simulink model "c00019M_harness"  (R2018a)
settings: Solver=ode3  StartTime=0.0  StopTime=10.0  RelTol=1e-3  EnableMultiTasking=on
undefined symbols (not defined in the file): b, DiscIntNeverNeededParam, J, K, L, PosMinimaW4, R, sigbuilder_block
(part 2 of 3)

== system c00019M_harness/CPSUT/Cyber/WL1 ==
  note: Sensors
  WPos : Inport
  User : Inport  Port=2
  OW : Inport  Port=3
  Chart1 : Stateflow chart  TreatAsAtomicUnit=on
  Constant : Constant  Value=-1
  Data Type Conversion : DataTypeConversion
  Switch : Switch  Criteria=u2 ~= 0  Threshold=1  ZeroCross=off
  WindowLogicOutput : Outport
  wires:
  Data Type Conversion/1 -> Switch/2
  Constant/1 -> Switch/1
  User/1 -> Chart1/2(UI)
  WPos/1 -> Chart1/1(S)
  Switch/1 -> WindowLogicOutput/1
  OW/1 -> Data Type Conversion/1
  Chart1/1(W) -> Switch/3

== system c00019M_harness/CPSUT/Cyber/WL3 ==
  note: Sensors
  WPos : Inport
  User : Inport  Port=2
  OW : Inport  Port=3
  L : Inport  Port=4
  Chart2 : Stateflow chart  TreatAsAtomicUnit=on
  Constant : Constant  Value=-1
  Constant1 : Constant  Value=0
  Constant2 : Constant  Value=PosMinimaW4
  Data Type Conversion : DataTypeConversion
  Switch : Switch  Criteria=u2 ~= 0  Threshold=1  ZeroCross=off
  Switch1 : Switch  Criteria=u2 ~= 0
  WindowLogicOutput : Outport
  wires:
  L/1 -> Switch1/2
  Data Type Conversion/1 -> Switch/2
  Constant/1 -> Switch/1
  Chart2/1(W) -> Switch1/3
  User/1 -> Chart2/2(UI)
  WPos/1 -> Chart2/1(S)
  Switch1/1 -> Switch/3
  Constant1/1 -> Switch1/1
  Switch/1 -> WindowLogicOutput/1
  OW/1 -> Data Type Conversion/1
  Constant2/1 -> Chart2/3(PosMinW4)

== system c00019M_harness/CPSUT/Physical/W ==
  WIn : Inport
  DC_Engine : Subsystem
  Discrete-Time Integrator : DiscreteIntegrator  InitialCondition=5  SampleTime=-1  LimitOutput=on  UpperSaturationLimit=5  LowerSaturationLimit=0  ICPrevOutput=DiscIntNeverNeededParam  ICPrevScaledInput=DiscIntNeverNeededParam
  WPos : Outport
  wires:
  Discrete-Time Integrator/1 -> WPos/1
  DC_Engine/1(Speed) -> Discrete-Time Integrator/1
  WIn/1 -> DC_Engine/1(input)

== system c00019M_harness/CPSUT/Physical/W5 ==
  WIn : Inport
  DC_Engine : Subsystem
  Discrete-Time Integrator : DiscreteIntegrator  InitialCondition=5  SampleTime=-1  LimitOutput=on  UpperSaturationLimit=5  LowerSaturationLimit=0  ICPrevOutput=DiscIntNeverNeededParam  ICPrevScaledInput=DiscIntNeverNeededParam
  WPos : Outport
  wires:
  WIn/1 -> DC_Engine/1(input)
  DC_Engine/1(Speed) -> Discrete-Time Integrator/1
  Discrete-Time Integrator/1 -> WPos/1

== system c00019M_harness/CPSUT/Physical/W7 ==
  WIn : Inport
  DC_Engine : Subsystem
  Discrete-Time Integrator : DiscreteIntegrator  InitialCondition=5  SampleTime=-1  LimitOutput=on  UpperSaturationLimit=5  LowerSaturationLimit=PosMinimaW4  ICPrevOutput=DiscIntNeverNeededParam  ICPrevScaledInput=DiscIntNeverNeededParam
  WPos : Outport
  wires:
  WIn/1 -> DC_Engine/1(input)
  DC_Engine/1(Speed) -> Discrete-Time Integrator/1
  Discrete-Time Integrator/1 -> WPos/1

== system c00019M_harness/M004/Cyber/Pri ==
  P : Inport
  CW2C : Inport  Port=2
  Switch1 : Switch  Criteria=u2 > Threshold  Threshold=4
  User : Outport
  wires:
  CW2C/1 -> Switch1/3
  P/1 -> Switch1/1, Switch1/2
  Switch1/1 -> User/1

== system c00019M_harness/M004/Cyber/Pri3 ==
  D : Inport
  CW1C : Inport  Port=2
  Switch : Switch  Criteria=u2 ~= 0
  User : Outport
  wires:
  D/1 -> Switch/1, Switch/2
  Switch/1 -> User/1
  CW1C/1 -> Switch/3

== system c00019M_harness/M004/Cyber/Pri4 ==
  P : Inport
  CW4C : Inport  Port=2
  Switch1 : Switch  Criteria=u2 ~= 0
  User : Outport
  wires:
  P/1 -> Switch1/1, Switch1/2
  CW4C/1 -> Switch1/3
  Switch1/1 -> User/1

== system c00019M_harness/M004/Cyber/WL ==
  note: Sensors
  WPos : Inport
  User : Inport  Port=2
  OW : Inport  Port=3
  Chart : Stateflow chart  TreatAsAtomicUnit=on
  Constant : Constant  Value=-1
  Data Type Conversion : DataTypeConversion
  Switch : Switch  Criteria=u2 ~= 0  Threshold=1  ZeroCross=off
  WindowLogicOutput : Outport
  wires:
  Data Type Conversion/1 -> Switch/2
  Constant/1 -> Switch/1
  User/1 -> Chart/2(UI)
  WPos/1 -> Chart/1(S)
  Switch/1 -> WindowLogicOutput/1
  OW/1 -> Data Type Conversion/1
  Chart/1(W) -> Switch/3

== system c00019M_harness/M004/Cyber/WL1 ==
  note: Sensors
  WPos : Inport
  User : Inport  Port=2
  OW : Inport  Port=3
  Chart1 : Stateflow chart  TreatAsAtomicUnit=on
  Constant : Constant  Value=-1
  Data Type Conversion : DataTypeConversion
  Switch : Switch  Criteria=u2 ~= 0  Threshold=1  ZeroCross=off
  WindowLogicOutput : Outport
  wires:
  OW/1 -> Data Type Conversion/1
  Switch/1 -> WindowLogicOutput/1
  WPos/1 -> Chart1/1(S)
  User/1 -> Chart1/2(UI)
  Constant/1 -> Switch/1
  Data Type Conversion/1 -> Switch/2
  Chart1/1(W) -> Switch/3

== system c00019M_harness/M004/Cyber/WL3 ==
  note: Sensors
  WPos : Inport
  User : Inport  Port=2
  OW : Inport  Port=3
  L : Inport  Port=4
  Chart2 : Stateflow chart  TreatAsAtomicUnit=on
  Constant : Constant  Value=-1
  Constant1 : Constant  Value=0
  Constant2 : Constant  Value=PosMinimaW4
  Data Type Conversion : DataTypeConversion
  Switch : Switch  Criteria=u2 ~= 0  Threshold=1  ZeroCross=off
  Switch1 : Switch  Criteria=u2 ~= 0
  WindowLogicOutput : Outport
  wires:
  Constant2/1 -> Chart2/3(PosMinW4)
  OW/1 -> Data Type Conversion/1
  Switch/1 -> WindowLogicOutput/1
  Constant1/1 -> Switch1/1
  Switch1/1 -> Switch/3
  WPos/1 -> Chart2/1(S)
  User/1 -> Chart2/2(UI)
  Chart2/1(W) -> Switch1/3
  Constant/1 -> Switch/1
  Data Type Conversion/1 -> Switch/2
  L/1 -> Switch1/2

== system c00019M_harness/M004/Physical/W ==
  WIn : Inport
  DC_Engine : Subsystem
  Discrete-Time Integrator : DiscreteIntegrator  InitialCondition=5  SampleTime=-1  LimitOutput=on  UpperSaturationLimit=5  LowerSaturationLimit=0  ICPrevOutput=DiscIntNeverNeededParam  ICPrevScaledInput=DiscIntNeverNeededParam
  WPos : Outport
  wires:
  WIn/1 -> DC_Engine/1(input)
  DC_Engine/1(Speed) -> Discrete-Time Integrator/1
  Discrete-Time Integrator/1 -> WPos/1

== system c00019M_harness/M004/Physical/W5 ==
  WIn : Inport
  DC_Engine : Subsystem
  Discrete-Time Integrator : DiscreteIntegrator  InitialCondition=5  SampleTime=-1  LimitOutput=on  UpperSaturationLimit=5  LowerSaturationLimit=0  ICPrevOutput=DiscIntNeverNeededParam  ICPrevScaledInput=DiscIntNeverNeededParam
  WPos : Outport
  wires:
  Discrete-Time Integrator/1 -> WPos/1
  DC_Engine/1(Speed) -> Discrete-Time Integrator/1
  WIn/1 -> DC_Engine/1(input)

== system c00019M_harness/M004/Physical/W7 ==
  WIn : Inport
  DC_Engine : Subsystem
  Discrete-Time Integrator : DiscreteIntegrator  InitialCondition=5  SampleTime=-1  LimitOutput=on  UpperSaturationLimit=5  LowerSaturationLimit=PosMinimaW4  ICPrevOutput=DiscIntNeverNeededParam  ICPrevScaledInput=DiscIntNeverNeededParam
  WPos : Outport
  wires:
  Discrete-Time Integrator/1 -> WPos/1
  DC_Engine/1(Speed) -> Discrete-Time Integrator/1
  WIn/1 -> DC_Engine/1(input)

== system c00019M_harness/M014/Cyber/Pri ==
  P : Inport
  CW2C : Inport  Port=2
  Switch1 : Switch  Criteria=u2 ~= 0
  User : Outport
  wires:
  CW2C/1 -> Switch1/3
  P/1 -> Switch1/1, Switch1/2
  Switch1/1 -> User/1

== system c00019M_harness/M014/Cyber/Pri3 ==
  D : Inport
  CW1C : Inport  Port=2
  Switch : Switch  Criteria=u2 > Threshold  Threshold=4
  User : Outport
  wires:
  D/1 -> Switch/1, Switch/2
  Switch/1 -> User/1
  CW1C/1 -> Switch/3

== system c00019M_harness/M014/Cyber/Pri4 ==
  P : Inport
  CW4C : Inport  Port=2
  Switch1 : Switch  Criteria=u2 ~= 0
  User : Outport
  wires:
  P/1 -> Switch1/1, Switch1/2
  CW4C/1 -> Switch1/3
  Switch1/1 -> User/1

== system c00019M_harness/M014/Cyber/WL ==
  note: Sensors
  WPos : Inport
  User : Inport  Port=2
  OW : Inport  Port=3
  Chart : Stateflow chart  TreatAsAtomicUnit=on
  Constant : Constant  Value=-1
  Data Type Conversion : DataTypeConversion
  Switch : Switch  Criteria=u2 ~= 0  Threshold=1  ZeroCross=off
  WindowLogicOutput : Outport
  wires:
  Data Type Conversion/1 -> Switch/2
  Constant/1 -> Switch/1
  User/1 -> Chart/2(UI)
  WPos/1 -> Chart/1(S)
  Switch/1 -> WindowLogicOutput/1
  OW/1 -> Data Type Conversion/1
  Chart/1(W) -> Switch/3

== system c00019M_harness/M014/Cyber/WL1 ==
  note: Sensors
  WPos : Inport
  User : Inport  Port=2
  OW : Inport  Port=3
  Chart1 : Stateflow chart  TreatAsAtomicUnit=on
  Constant : Constant  Value=-1
  Data Type Conversion : DataTypeConversion
  Switch : Switch  Criteria=u2 ~= 0  Threshold=1  ZeroCross=off
  WindowLogicOutput : Outport
  wires:
  OW/1 -> Data Type Conversion/1
  Switch/1 -> WindowLogicOutput/1
  WPos/1 -> Chart1/1(S)
  User/1 -> Chart1/2(UI)
  Constant/1 -> Switch/1
  Data Type Conversion/1 -> Switch/2
  Chart1/1(W) -> Switch/3

== system c00019M_harness/M014/Cyber/WL3 ==
  note: Sensors
  WPos : Inport
  User : Inport  Port=2
  OW : Inport  Port=3
  L : Inport  Port=4
  Chart2 : Stateflow chart  TreatAsAtomicUnit=on
  Constant : Constant  Value=-1
  Constant1 : Constant  Value=0
  Constant2 : Constant  Value=PosMinimaW4
  Data Type Conversion : DataTypeConversion
  Switch : Switch  Criteria=u2 ~= 0  Threshold=1  ZeroCross=off
  Switch1 : Switch  Criteria=u2 ~= 0
  WindowLogicOutput : Outport
  wires:
  Constant2/1 -> Chart2/3(PosMinW4)
  OW/1 -> Data Type Conversion/1
  Switch/1 -> WindowLogicOutput/1
  Constant1/1 -> Switch1/1
  Switch1/1 -> Switch/3
  WPos/1 -> Chart2/1(S)
  User/1 -> Chart2/2(UI)
  Chart2/1(W) -> Switch1/3
  Constant/1 -> Switch/1
  Data Type Conversion/1 -> Switch/2
  L/1 -> Switch1/2

== system c00019M_harness/M014/Physical/W ==
  WIn : Inport
  DC_Engine : Subsystem
  Discrete-Time Integrator : DiscreteIntegrator  InitialCondition=5  SampleTime=-1  LimitOutput=on  UpperSaturationLimit=5  LowerSaturationLimit=0  ICPrevOutput=DiscIntNeverNeededParam  ICPrevScaledInput=DiscIntNeverNeededParam
  WPos : Outport
  wires:
  WIn/1 -> DC_Engine/1(input)
  DC_Engine/1(Speed) -> Discrete-Time Integrator/1
  Discrete-Time Integrator/1 -> WPos/1

== system c00019M_harness/M014/Physical/W5 ==
  WIn : Inport
  DC_Engine : Subsystem
  Discrete-Time Integrator : DiscreteIntegrator  InitialCondition=5  SampleTime=-1  LimitOutput=on  UpperSaturationLimit=5  LowerSaturationLimit=0  ICPrevOutput=DiscIntNeverNeededParam  ICPrevScaledInput=DiscIntNeverNeededParam
  WPos : Outport
  wires:
  Discrete-Time Integrator/1 -> WPos/1
  DC_Engine/1(Speed) -> Discrete-Time Integrator/1
  WIn/1 -> DC_Engine/1(input)

== system c00019M_harness/M014/Physical/W7 ==
  WIn : Inport
  DC_Engine : Subsystem
  Discrete-Time Integrator : DiscreteIntegrator  InitialCondition=5  SampleTime=-1  LimitOutput=on  UpperSaturationLimit=5  LowerSaturationLimit=PosMinimaW4  ICPrevOutput=DiscIntNeverNeededParam  ICPrevScaledInput=DiscIntNeverNeededParam
  WPos : Outport
  wires:
  Discrete-Time Integrator/1 -> WPos/1
  DC_Engine/1(Speed) -> Discrete-Time Integrator/1
  WIn/1 -> DC_Engine/1(input)

== system c00019M_harness/M018/Cyber/Pri ==
  P : Inport
  CW2C : Inport  Port=2
  Switch1 : Switch  Criteria=u2 ~= 0
  User : Outport
  wires:
  CW2C/1 -> Switch1/3
  P/1 -> Switch1/1, Switch1/2
  Switch1/1 -> User/1

== system c00019M_harness/M018/Cyber/Pri3 ==
  D : Inport
  CW1C : Inport  Port=2
  Switch : Switch  Criteria=u2 ~= 0
  User : Outport
  wires:
  D/1 -> Switch/1, Switch/2
  Switch/1 -> User/1
  CW1C/1 -> Switch/3

== system c00019M_harness/M018/Cyber/Pri4 ==
  P : Inport
  CW4C : Inport  Port=2
  Switch1 : Switch  Criteria=u2 > Threshold  Threshold=4
  User : Outport
  wires:
  P/1 -> Switch1/1, Switch1/2
  CW4C/1 -> Switch1/3
  Switch1/1 -> User/1

== system c00019M_harness/M018/Cyber/WL ==
  note: Sensors
  WPos : Inport
  User : Inport  Port=2
  OW : Inport  Port=3
  Chart : Stateflow chart  TreatAsAtomicUnit=on
  Constant : Constant  Value=-1
  Data Type Conversion : DataTypeConversion
  Switch : Switch  Criteria=u2 ~= 0  Threshold=1  ZeroCross=off
  WindowLogicOutput : Outport
  wires:
  Data Type Conversion/1 -> Switch/2
  Constant/1 -> Switch/1
  User/1 -> Chart/2(UI)
  WPos/1 -> Chart/1(S)
  Switch/1 -> WindowLogicOutput/1
  OW/1 -> Data Type Conversion/1
  Chart/1(W) -> Switch/3

== system c00019M_harness/M018/Cyber/WL1 ==
  note: Sensors
  WPos : Inport
  User : Inport  Port=2
  OW : Inport  Port=3
  Chart1 : Stateflow chart  TreatAsAtomicUnit=on
  Constant : Constant  Value=-1
  Data Type Conversion : DataTypeConversion
  Switch : Switch  Criteria=u2 ~= 0  Threshold=1  ZeroCross=off
  WindowLogicOutput : Outport
  wires:
  OW/1 -> Data Type Conversion/1
  Switch/1 -> WindowLogicOutput/1
  WPos/1 -> Chart1/1(S)
  User/1 -> Chart1/2(UI)
  Constant/1 -> Switch/1
  Data Type Conversion/1 -> Switch/2
  Chart1/1(W) -> Switch/3

== system c00019M_harness/M018/Cyber/WL3 ==
  note: Sensors
  WPos : Inport
  User : Inport  Port=2
  OW : Inport  Port=3
  L : Inport  Port=4
  Chart2 : Stateflow chart  TreatAsAtomicUnit=on
  Constant : Constant  Value=-1
  Constant1 : Constant  Value=0
  Constant2 : Constant  Value=PosMinimaW4
  Data Type Conversion : DataTypeConversion
  Switch : Switch  Criteria=u2 ~= 0  Threshold=1  ZeroCross=off
  Switch1 : Switch  Criteria=u2 ~= 0
  WindowLogicOutput : Outport
  wires:
  Constant2/1 -> Chart2/3(PosMinW4)
  OW/1 -> Data Type Conversion/1
  Switch/1 -> WindowLogicOutput/1
  Constant1/1 -> Switch1/1
  Switch1/1 -> Switch/3
  WPos/1 -> Chart2/1(S)
  User/1 -> Chart2/2(UI)
  Chart2/1(W) -> Switch1/3
  Constant/1 -> Switch/1
  Data Type Conversion/1 -> Switch/2
  L/1 -> Switch1/2

== system c00019M_harness/M018/Physical/W ==
  WIn : Inport
  DC_Engine : Subsystem
  Discrete-Time Integrator : DiscreteIntegrator  InitialCondition=5  SampleTime=-1  LimitOutput=on  UpperSaturationLimit=5  LowerSaturationLimit=0  ICPrevOutput=DiscIntNeverNeededParam  ICPrevScaledInput=DiscIntNeverNeededParam
  WPos : Outport
  wires:
  WIn/1 -> DC_Engine/1(input)
  DC_Engine/1(Speed) -> Discrete-Time Integrator/1
  Discrete-Time Integrator/1 -> WPos/1

== system c00019M_harness/M018/Physical/W5 ==
  WIn : Inport
  DC_Engine : Subsystem
  Discrete-Time Integrator : DiscreteIntegrator  InitialCondition=5  SampleTime=-1  LimitOutput=on  UpperSaturationLimit=5  LowerSaturationLimit=0  ICPrevOutput=DiscIntNeverNeededParam  ICPrevScaledInput=DiscIntNeverNeededParam
  WPos : Outport
  wires:
  Discrete-Time Integrator/1 -> WPos/1
  DC_Engine/1(Speed) -> Discrete-Time Integrator/1
  WIn/1 -> DC_Engine/1(input)

== system c00019M_harness/M018/Physical/W7 ==
  WIn : Inport
  DC_Engine : Subsystem
  Discrete-Time Integrator : DiscreteIntegrator  InitialCondition=5  SampleTime=-1  LimitOutput=on  UpperSaturationLimit=5  LowerSaturationLimit=PosMinimaW4  ICPrevOutput=DiscIntNeverNeededParam  ICPrevScaledInput=DiscIntNeverNeededParam
  WPos : Outport
  wires:
  Discrete-Time Integrator/1 -> WPos/1
  DC_Engine/1(Speed) -> Discrete-Time Integrator/1
  WIn/1 -> DC_Engine/1(input)

== system c00019M_harness/M028/Cyber/Pri ==
  P : Inport
  CW2C : Inport  Port=2
  Switch1 : Switch  Criteria=u2 ~= 0
  User : Outport
  wires:
  CW2C/1 -> Switch1/3
  P/1 -> Switch1/1, Switch1/2
  Switch1/1 -> User/1

== system c00019M_harness/M028/Cyber/Pri3 ==
  D : Inport
  CW1C : Inport  Port=2
  Switch : Switch  Criteria=u2 ~= 0
  User : Outport
  wires:
  D/1 -> Switch/1, Switch/2
  Switch/1 -> User/1
  CW1C/1 -> Switch/3

== system c00019M_harness/M028/Cyber/Pri4 ==
  P : Inport
  CW4C : Inport  Port=2
  Switch1 : Switch  Criteria=u2 ~= 0
  User : Outport
  wires:
  P/1 -> Switch1/1, Switch1/2
  CW4C/1 -> Switch1/3
  Switch1/1 -> User/1

== system c00019M_harness/M028/Cyber/WL ==
  note: Sensors
  WPos : Inport
  User : Inport  Port=2
  OW : Inport  Port=3
  Chart : Stateflow chart  TreatAsAtomicUnit=on
  Constant : Constant  Value=-1
  Data Type Conversion : DataTypeConversion
  Switch : Switch  Criteria=u2 ~= 0  Threshold=1  ZeroCross=off
  WindowLogicOutput : Outport
  wires:
  Data Type Conversion/1 -> Switch/2
  Constant/1 -> Switch/1
  User/1 -> Chart/2(UI)
  WPos/1 -> Chart/1(S)
  Switch/1 -> WindowLogicOutput/1
  OW/1 -> Data Type Conversion/1
  Chart/1(W) -> Switch/3

== system c00019M_harness/M028/Cyber/WL1 ==
  note: Sensors
  WPos : Inport
  User : Inport  Port=2
  OW : Inport  Port=3
  Chart1 : Stateflow chart  TreatAsAtomicUnit=on
  Constant : Constant  Value=-1
  Data Type Conversion : DataTypeConversion
  Switch : Switch  Criteria=u2 ~= 0  Threshold=1  ZeroCross=off
  WindowLogicOutput : Outport
  wires:
  OW/1 -> Data Type Conversion/1
  Switch/1 -> WindowLogicOutput/1
  WPos/1 -> Chart1/1(S)
  User/1 -> Chart1/2(UI)
  Constant/1 -> Switch/1
  Data Type Conversion/1 -> Switch/2
  Chart1/1(W) -> Switch/3

== system c00019M_harness/M028/Cyber/WL3 ==
  note: Sensors
  WPos : Inport
  User : Inport  Port=2
  OW : Inport  Port=3
  L : Inport  Port=4
  Chart2 : Stateflow chart  TreatAsAtomicUnit=on
  Constant : Constant  Value=-1
  Constant1 : Constant  Value=0
  Constant2 : Constant  Value=PosMinimaW4
  Data Type Conversion : DataTypeConversion
  Switch : Switch  Criteria=u2 ~= 0  Threshold=1  ZeroCross=off
  Switch1 : Switch  Criteria=u2 > Threshold  Threshold=4
  WindowLogicOutput : Outport
  wires:
  Constant2/1 -> Chart2/3(PosMinW4)
  OW/1 -> Data Type Conversion/1
  Switch/1 -> WindowLogicOutput/1
  Constant1/1 -> Switch1/1
  Switch1/1 -> Switch/3
  WPos/1 -> Chart2/1(S)
  User/1 -> Chart2/2(UI)
  Chart2/1(W) -> Switch1/3
  Constant/1 -> Switch/1
  Data Type Conversion/1 -> Switch/2
  L/1 -> Switch1/2

== system c00019M_harness/M028/Physical/W ==
  WIn : Inport
  DC_Engine : Subsystem
  Discrete-Time Integrator : DiscreteIntegrator  InitialCondition=5  SampleTime=-1  LimitOutput=on  UpperSaturationLimit=5  LowerSaturationLimit=0  ICPrevOutput=DiscIntNeverNeededParam  ICPrevScaledInput=DiscIntNeverNeededParam
  WPos : Outport
  wires:
  WIn/1 -> DC_Engine/1(input)
  DC_Engine/1(Speed) -> Discrete-Time Integrator/1
  Discrete-Time Integrator/1 -> WPos/1

== system c00019M_harness/M028/Physical/W5 ==
  WIn : Inport
  DC_Engine : Subsystem
  Discrete-Time Integrator : DiscreteIntegrator  InitialCondition=5  SampleTime=-1  LimitOutput=on  UpperSaturationLimit=5  LowerSaturationLimit=0  ICPrevOutput=DiscIntNeverNeededParam  ICPrevScaledInput=DiscIntNeverNeededParam
  WPos : Outport
  wires:
  Discrete-Time Integrator/1 -> WPos/1
  DC_Engine/1(Speed) -> Discrete-Time Integrator/1
  WIn/1 -> DC_Engine/1(input)

== system c00019M_harness/M028/Physical/W7 ==
  WIn : Inport
  DC_Engine : Subsystem
  Discrete-Time Integrator : DiscreteIntegrator  InitialCondition=5  SampleTime=-1  LimitOutput=on  UpperSaturationLimit=5  LowerSaturationLimit=PosMinimaW4  ICPrevOutput=DiscIntNeverNeededParam  ICPrevScaledInput=DiscIntNeverNeededParam
  WPos : Outport
  wires:
  Discrete-Time Integrator/1 -> WPos/1
  DC_Engine/1(Speed) -> Discrete-Time Integrator/1
  WIn/1 -> DC_Engine/1(input)

== system c00019M_harness/M033/Cyber/Pri ==
  P : Inport
  CW2C : Inport  Port=2
  Switch1 : Switch  Criteria=u2 ~= 0
  User : Outport
  wires:
  CW2C/1 -> Switch1/2, Switch1/1
  P/1 -> Switch1/3
  Switch1/1 -> User/1

== system c00019M_harness/M033/Cyber/Pri3 ==
  D : Inport
  CW1C : Inport  Port=2
  Switch : Switch  Criteria=u2 ~= 0
  User : Outport
  wires:
  D/1 -> Switch/1, Switch/2
  Switch/1 -> User/1
  CW1C/1 -> Switch/3

== system c00019M_harness/M033/Cyber/Pri4 ==
  P : Inport
  CW4C : Inport  Port=2
  Switch1 : Switch  Criteria=u2 ~= 0
  User : Outport
  wires:
  P/1 -> Switch1/1, Switch1/2
  CW4C/1 -> Switch1/3
  Switch1/1 -> User/1

== system c00019M_harness/M033/Cyber/WL ==
  note: Sensors
  WPos : Inport
  User : Inport  Port=2
  OW : Inport  Port=3
  Chart : Stateflow chart  TreatAsAtomicUnit=on
  Constant : Constant  Value=-1
  Data Type Conversion : DataTypeConversion
  Switch : Switch  Criteria=u2 ~= 0  Threshold=1  ZeroCross=off
  WindowLogicOutput : Outport
  wires:
  Data Type Conversion/1 -> Switch/2
  Constant/1 -> Switch/1
  User/1 -> Chart/2(UI)
  WPos/1 -> Chart/1(S)
  Switch/1 -> WindowLogicOutput/1
  OW/1 -> Data Type Conversion/1
  Chart/1(W) -> Switch/3

== system c00019M_harness/M033/Cyber/WL1 ==
  note: Sensors
  WPos : Inport
  User : Inport  Port=2
  OW : Inport  Port=3
  Chart1 : Stateflow chart  TreatAsAtomicUnit=on
  Constant : Constant  Value=-1
  Data Type Conversion : DataTypeConversion
  Switch : Switch  Criteria=u2 ~= 0  Threshold=1  ZeroCross=off
  WindowLogicOutput : Outport
  wires:
  OW/1 -> Data Type Conversion/1
  Switch/1 -> WindowLogicOutput/1
  WPos/1 -> Chart1/1(S)
  User/1 -> Chart1/2(UI)
  Constant/1 -> Switch/1
  Data Type Conversion/1 -> Switch/2
  Chart1/1(W) -> Switch/3

== system c00019M_harness/M033/Cyber/WL3 ==
  note: Sensors
  WPos : Inport
  User : Inport  Port=2
  OW : Inport  Port=3
  L : Inport  Port=4
  Chart2 : Stateflow chart  TreatAsAtomicUnit=on
  Constant : Constant  Value=-1
  Constant1 : Constant  Value=0
  Constant2 : Constant  Value=PosMinimaW4
  Data Type Conversion : DataTypeConversion
  Switch : Switch  Criteria=u2 ~= 0  Threshold=1  ZeroCross=off
  Switch1 : Switch  Criteria=u2 ~= 0
  WindowLogicOutput : Outport
  wires:
  Constant2/1 -> Chart2/3(PosMinW4)
  OW/1 -> Data Type Conversion/1
  Switch/1 -> WindowLogicOutput/1
  Constant1/1 -> Switch1/1
  Switch1/1 -> Switch/3
  WPos/1 -> Chart2/1(S)
  User/1 -> Chart2/2(UI)
  Chart2/1(W) -> Switch1/3
  Constant/1 -> Switch/1
  Data Type Conversion/1 -> Switch/2
  L/1 -> Switch1/2

== system c00019M_harness/M033/Physical/W ==
  WIn : Inport
  DC_Engine : Subsystem
  Discrete-Time Integrator : DiscreteIntegrator  InitialCondition=5  SampleTime=-1  LimitOutput=on  UpperSaturationLimit=5  LowerSaturationLimit=0  ICPrevOutput=DiscIntNeverNeededParam  ICPrevScaledInput=DiscIntNeverNeededParam
  WPos : Outport
  wires:
  WIn/1 -> DC_Engine/1(input)
  DC_Engine/1(Speed) -> Discrete-Time Integrator/1
  Discrete-Time Integrator/1 -> WPos/1

== system c00019M_harness/M033/Physical/W5 ==
  WIn : Inport
  DC_Engine : Subsystem
  Discrete-Time Integrator : DiscreteIntegrator  InitialCondition=5  SampleTime=-1  LimitOutput=on  UpperSaturationLimit=5  LowerSaturationLimit=0  ICPrevOutput=DiscIntNeverNeededParam  ICPrevScaledInput=DiscIntNeverNeededParam
  WPos : Outport
  wires:
  Discrete-Time Integrator/1 -> WPos/1
  DC_Engine/1(Speed) -> Discrete-Time Integrator/1
  WIn/1 -> DC_Engine/1(input)

== system c00019M_harness/M033/Physical/W7 ==
  WIn : Inport
  DC_Engine : Subsystem
  Discrete-Time Integrator : DiscreteIntegrator  InitialCondition=5  SampleTime=-1  LimitOutput=on  UpperSaturationLimit=5  LowerSaturationLimit=PosMinimaW4  ICPrevOutput=DiscIntNeverNeededParam  ICPrevScaledInput=DiscIntNeverNeededParam
  WPos : Outport
  wires:
  Discrete-Time Integrator/1 -> WPos/1
  DC_Engine/1(Speed) -> Discrete-Time Integrator/1
  WIn/1 -> DC_Engine/1(input)

== system c00019M_harness/M043/Cyber/Pri ==
  P : Inport
  CW2C : Inport  Port=2
  Switch1 : Switch  Criteria=u2 ~= 0
  User : Outport
  wires:
  CW2C/1 -> Switch1/3
  P/1 -> Switch1/1, Switch1/2
  Switch1/1 -> User/1

== system c00019M_harness/M043/Cyber/Pri3 ==
  D : Inport
  CW1C : Inport  Port=2
  Switch : Switch  Criteria=u2 ~= 0
  User : Outport
  wires:
  Switch/1 -> User/1
  CW1C/1 -> Switch/2, Switch/1
  D/1 -> Switch/3

== system c00019M_harness/M043/Cyber/Pri4 ==
  P : Inport
  CW4C : Inport  Port=2
  Switch1 : Switch  Criteria=u2 ~= 0
  User : Outport
  wires:
  P/1 -> Switch1/1, Switch1/2
  CW4C/1 -> Switch1/3
  Switch1/1 -> User/1

== system c00019M_harness/M043/Cyber/WL ==
  note: Sensors
  WPos : Inport
  User : Inport  Port=2
  OW : Inport  Port=3
  Chart : Stateflow chart  TreatAsAtomicUnit=on
  Constant : Constant  Value=-1
  Data Type Conversion : DataTypeConversion
  Switch : Switch  Criteria=u2 ~= 0  Threshold=1  ZeroCross=off
  WindowLogicOutput : Outport
  wires:
  Data Type Conversion/1 -> Switch/2
  Constant/1 -> Switch/1
  User/1 -> Chart/2(UI)
  WPos/1 -> Chart/1(S)
  Switch/1 -> WindowLogicOutput/1
  OW/1 -> Data Type Conversion/1
  Chart/1(W) -> Switch/3

== system c00019M_harness/M043/Cyber/WL1 ==
  note: Sensors
  WPos : Inport
  User : Inport  Port=2
  OW : Inport  Port=3
  Chart1 : Stateflow chart  TreatAsAtomicUnit=on
  Constant : Constant  Value=-1
  Data Type Conversion : DataTypeConversion
  Switch : Switch  Criteria=u2 ~= 0  Threshold=1  ZeroCross=off
  WindowLogicOutput : Outport
  wires:
  OW/1 -> Data Type Conversion/1
  Switch/1 -> WindowLogicOutput/1
  WPos/1 -> Chart1/1(S)
  User/1 -> Chart1/2(UI)
  Constant/1 -> Switch/1
  Data Type Conversion/1 -> Switch/2
  Chart1/1(W) -> Switch/3

== system c00019M_harness/M043/Cyber/WL3 ==
  note: Sensors
  WPos : Inport
  User : Inport  Port=2
  OW : Inport  Port=3
  L : Inport  Port=4
  Chart2 : Stateflow chart  TreatAsAtomicUnit=on
  Constant : Constant  Value=-1
  Constant1 : Constant  Value=0
  Constant2 : Constant  Value=PosMinimaW4
  Data Type Conversion : DataTypeConversion
  Switch : Switch  Criteria=u2 ~= 0  Threshold=1  ZeroCross=off
  Switch1 : Switch  Criteria=u2 ~= 0
  WindowLogicOutput : Outport
  wires:
  Constant2/1 -> Chart2/3(PosMinW4)
  OW/1 -> Data Type Conversion/1
  Switch/1 -> WindowLogicOutput/1
  Constant1/1 -> Switch1/1
  Switch1/1 -> Switch/3
  WPos/1 -> Chart2/1(S)
  User/1 -> Chart2/2(UI)
  Chart2/1(W) -> Switch1/3
  Constant/1 -> Switch/1
  Data Type Conversion/1 -> Switch/2
  L/1 -> Switch1/2

== system c00019M_harness/M043/Physical/W ==
  WIn : Inport
  DC_Engine : Subsystem
  Discrete-Time Integrator : DiscreteIntegrator  InitialCondition=5  SampleTime=-1  LimitOutput=on  UpperSaturationLimit=5  LowerSaturationLimit=0  ICPrevOutput=DiscIntNeverNeededParam  ICPrevScaledInput=DiscIntNeverNeededParam
  WPos : Outport
  wires:
  WIn/1 -> DC_Engine/1(input)
  DC_Engine/1(Speed) -> Discrete-Time Integrator/1
  Discrete-Time Integrator/1 -> WPos/1

== system c00019M_harness/M043/Physical/W5 ==
  WIn : Inport
  DC_Engine : Subsystem
  Discrete-Time Integrator : DiscreteIntegrator  InitialCondition=5  SampleTime=-1  LimitOutput=on  UpperSaturationLimit=5  LowerSaturationLimit=0  ICPrevOutput=DiscIntNeverNeededParam  ICPrevScaledInput=DiscIntNeverNeededParam
  WPos : Outport
  wires:
  Discrete-Time Integrator/1 -> WPos/1
  DC_Engine/1(Speed) -> Discrete-Time Integrator/1
  WIn/1 -> DC_Engine/1(input)

== system c00019M_harness/M043/Physical/W7 ==
  WIn : Inport
  DC_Engine : Subsystem
  Discrete-Time Integrator : DiscreteIntegrator  InitialCondition=5  SampleTime=-1  LimitOutput=on  UpperSaturationLimit=5  LowerSaturationLimit=PosMinimaW4  ICPrevOutput=DiscIntNeverNeededParam  ICPrevScaledInput=DiscIntNeverNeededParam
  WPos : Outport
  wires:
  Discrete-Time Integrator/1 -> WPos/1
  DC_Engine/1(Speed) -> Discrete-Time Integrator/1
  WIn/1 -> DC_Engine/1(input)

== system c00019M_harness/M047/Cyber/Pri ==
  P : Inport
  CW2C : Inport  Port=2
  Switch1 : Switch  Criteria=u2 ~= 0
  User : Outport
  wires:
  CW2C/1 -> Switch1/3
  P/1 -> Switch1/1, Switch1/2
  Switch1/1 -> User/1

== system c00019M_harness/M047/Cyber/Pri3 ==
  D : Inport
  CW1C : Inport  Port=2
  Switch : Switch  Criteria=u2 ~= 0
  User : Outport
  wires:
  D/1 -> Switch/1, Switch/2
  Switch/1 -> User/1
  CW1C/1 -> Switch/3

== system c00019M_harness/M047/Cyber/Pri4 ==
  P : Inport
  CW4C : Inport  Port=2
  Switch1 : Switch  Criteria=u2 ~= 0
  User : Outport
  wires:
  P/1 -> Switch1/3
  CW4C/1 -> Switch1/1
  Switch1/1 -> User/1

== system c00019M_harness/M047/Cyber/WL ==
  note: Sensors
  WPos : Inport
  User : Inport  Port=2
  OW : Inport  Port=3
  Chart : Stateflow chart  TreatAsAtomicUnit=on
  Constant : Constant  Value=-1
  Data Type Conversion : DataTypeConversion
  Switch : Switch  Criteria=u2 ~= 0  Threshold=1  ZeroCross=off
  WindowLogicOutput : Outport
  wires:
  Data Type Conversion/1 -> Switch/2
  Constant/1 -> Switch/1
  User/1 -> Chart/2(UI)
  WPos/1 -> Chart/1(S)
  Switch/1 -> WindowLogicOutput/1
  OW/1 -> Data Type Conversion/1
  Chart/1(W) -> Switch/3

== system c00019M_harness/M047/Cyber/WL1 ==
  note: Sensors
  WPos : Inport
  User : Inport  Port=2
  OW : Inport  Port=3
  Chart1 : Stateflow chart  TreatAsAtomicUnit=on
  Constant : Constant  Value=-1
  Data Type Conversion : DataTypeConversion
  Switch : Switch  Criteria=u2 ~= 0  Threshold=1  ZeroCross=off
  WindowLogicOutput : Outport
  wires:
  OW/1 -> Data Type Conversion/1
  Switch/1 -> WindowLogicOutput/1
  WPos/1 -> Chart1/1(S)
  User/1 -> Chart1/2(UI)
  Constant/1 -> Switch/1
  Data Type Conversion/1 -> Switch/2
  Chart1/1(W) -> Switch/3

== system c00019M_harness/M047/Cyber/WL3 ==
  note: Sensors
  WPos : Inport
  User : Inport  Port=2
  OW : Inport  Port=3
  L : Inport  Port=4
  Chart2 : Stateflow chart  TreatAsAtomicUnit=on
  Constant : Constant  Value=-1
  Constant1 : Constant  Value=0
  Constant2 : Constant  Value=PosMinimaW4
  Data Type Conversion : DataTypeConversion
  Switch : Switch  Criteria=u2 ~= 0  Threshold=1  ZeroCross=off
  Switch1 : Switch  Criteria=u2 ~= 0
  WindowLogicOutput : Outport
  wires:
  Constant2/1 -> Chart2/3(PosMinW4)
  OW/1 -> Data Type Conversion/1
  Switch/1 -> WindowLogicOutput/1
  Constant1/1 -> Switch1/1
  Switch1/1 -> Switch/3
  WPos/1 -> Chart2/1(S)
  User/1 -> Chart2/2(UI)
  Chart2/1(W) -> Switch1/3
  Constant/1 -> Switch/1
  Data Type Conversion/1 -> Switch/2
  L/1 -> Switch1/2

== system c00019M_harness/M047/Physical/W ==
  WIn : Inport
  DC_Engine : Subsystem
  Discrete-Time Integrator : DiscreteIntegrator  InitialCondition=5  SampleTime=-1  LimitOutput=on  UpperSaturationLimit=5  LowerSaturationLimit=0  ICPrevOutput=DiscIntNeverNeededParam  ICPrevScaledInput=DiscIntNeverNeededParam
  WPos : Outport
  wires:
  WIn/1 -> DC_Engine/1(input)
  DC_Engine/1(Speed) -> Discrete-Time Integrator/1
  Discrete-Time Integrator/1 -> WPos/1

== system c00019M_harness/M047/Physical/W5 ==
  WIn : Inport
  DC_Engine : Subsystem
  Discrete-Time Integrator : DiscreteIntegrator  InitialCondition=5  SampleTime=-1  LimitOutput=on  UpperSaturationLimit=5  LowerSaturationLimit=0  ICPrevOutput=DiscIntNeverNeededParam  ICPrevScaledInput=DiscIntNeverNeededParam
  WPos : Outport
  wires:
  Discrete-Time Integrator/1 -> WPos/1
  DC_Engine/1(Speed) -> Discrete-Time Integrator/1
  WIn/1 -> DC_Engine/1(input)

== system c00019M_harness/M047/Physical/W7 ==
  WIn : Inport
  DC_Engine : Subsystem
  Discrete-Time Integrator : DiscreteIntegrator  InitialCondition=5  SampleTime=-1  LimitOutput=on  UpperSaturationLimit=5  LowerSaturationLimit=PosMinimaW4  ICPrevOutput=DiscIntNeverNeededParam  ICPrevScaledInput=DiscIntNeverNeededParam
  WPos : Outport
  wires:
  Discrete-Time Integrator/1 -> WPos/1
  DC_Engine/1(Speed) -> Discrete-Time Integrator/1
  WIn/1 -> DC_Engine/1(input)

== system c00019M_harness/CPSUT/Physical/W/DC_Engine ==
  input : Inport
  (Inductance) : Gain  Gain=1/L
  (Inductance)1 : Gain  Gain=1/J
  Add : Sum  Inputs=-+-
  Add1 : Sum  Inputs=+-
  Damping : Gain  Gain=b
  Discrete-Time Integrator : DiscreteIntegrator  SampleTime=-1  ICPrevOutput=DiscIntNeverNeededParam  ICPrevScaledInput=DiscIntNeverNeededParam
  Discrete-Time Integrator1 : DiscreteIntegrator  SampleTime=-1  ICPrevOutput=DiscIntNeverNeededParam  ICPrevScaledInput=DiscIntNeverNeededParam
  Ke : Gain  Gain=K
  Kt : Gain  Gain=K
  Resistance : Gain  Gain=R
  Voltage : Gain  Gain=10
  Speed : Outport
  wires:
  input/1 -> Voltage/1
  Voltage/1 -> Add/2
  Add/1 -> (Inductance)/1
  Discrete-Time Integrator/1 -> Kt/1, Resistance/1
  Resistance/1 -> Add/1
  Ke/1 -> Add/3
  Kt/1 -> Add1/1
  Add1/1 -> (Inductance)1/1
  (Inductance)1/1 -> Discrete-Time Integrator1/1
  Discrete-Time Integrator1/1 -> Ke/1, Speed/1, Damping/1
  Damping/1 -> Add1/2
  (Inductance)/1 -> Discrete-Time Integrator/1

== system c00019M_harness/CPSUT/Physical/W5/DC_Engine ==
  input : Inport
  (Inductance) : Gain  Gain=1/L
  (Inductance)1 : Gain  Gain=1/J
  Add : Sum  Inputs=-+-
  Add1 : Sum  Inputs=+-
  Damping : Gain  Gain=b
  Discrete-Time Integrator : DiscreteIntegrator  SampleTime=-1  ICPrevOutput=DiscIntNeverNeededParam  ICPrevScaledInput=DiscIntNeverNeededParam
  Discrete-Time Integrator1 : DiscreteIntegrator  SampleTime=-1  ICPrevOutput=DiscIntNeverNeededParam  ICPrevScaledInput=DiscIntNeverNeededParam
  Ke : Gain  Gain=K
  Kt : Gain  Gain=K
  Resistance : Gain  Gain=R
  Voltage : Gain  Gain=10
  Speed : Outport
  wires:
  Damping/1 -> Add1/2
  Discrete-Time Integrator1/1 -> Damping/1, Speed/1, Ke/1
  (Inductance)1/1 -> Discrete-Time Integrator1/1
  Add1/1 -> (Inductance)1/1
  Kt/1 -> Add1/1
  Ke/1 -> Add/3
  Resistance/1 -> Add/1
  Discrete-Time Integrator/1 -> Resistance/1, Kt/1
  (Inductance)/1 -> Discrete-Time Integrator/1
  Add/1 -> (Inductance)/1
  Voltage/1 -> Add/2
  input/1 -> Voltage/1

== system c00019M_harness/CPSUT/Physical/W7/DC_Engine ==
  input : Inport
  (Inductance) : Gain  Gain=1/L
  (Inductance)1 : Gain  Gain=1/J
  Add : Sum  Inputs=-+-
  Add1 : Sum  Inputs=+-
  Damping : Gain  Gain=b
  Discrete-Time Integrator : DiscreteIntegrator  SampleTime=-1  ICPrevOutput=DiscIntNeverNeededParam  ICPrevScaledInput=DiscIntNeverNeededParam
  Discrete-Time Integrator1 : DiscreteIntegrator  SampleTime=-1  ICPrevOutput=DiscIntNeverNeededParam  ICPrevScaledInput=DiscIntNeverNeededParam
  Ke : Gain  Gain=K
  Kt : Gain  Gain=K
  Resistance : Gain  Gain=R
  Voltage : Gain  Gain=10
  Speed : Outport
  wires:
  Damping/1 -> Add1/2
  Discrete-Time Integrator1/1 -> Damping/1, Speed/1, Ke/1
  (Inductance)1/1 -> Discrete-Time Integrator1/1
  Add1/1 -> (Inductance)1/1
  Kt/1 -> Add1/1
  Ke/1 -> Add/3
  Resistance/1 -> Add/1
  Discrete-Time Integrator/1 -> Resistance/1, Kt/1
  (Inductance)/1 -> Discrete-Time Integrator/1
  Add/1 -> (Inductance)/1
  Voltage/1 -> Add/2
  input/1 -> Voltage/1

== system c00019M_harness/M004/Physical/W/DC_Engine ==
  input : Inport
  (Inductance) : Gain  Gain=1/L
  (Inductance)1 : Gain  Gain=1/J
  Add : Sum  Inputs=-+-
  Add1 : Sum  Inputs=+-
  Damping : Gain  Gain=b
  Discrete-Time Integrator : DiscreteIntegrator  SampleTime=-1  ICPrevOutput=DiscIntNeverNeededParam  ICPrevScaledInput=DiscIntNeverNeededParam
  Discrete-Time Integrator1 : DiscreteIntegrator  SampleTime=-1  ICPrevOutput=DiscIntNeverNeededParam  ICPrevScaledInput=DiscIntNeverNeededParam
  Ke : Gain  Gain=K
  Kt : Gain  Gain=K
  Resistance : Gain  Gain=R
  Voltage : Gain  Gain=10
  Speed : Outport
  wires:
  (Inductance)/1 -> Discrete-Time Integrator/1
  Damping/1 -> Add1/2
  Discrete-Time Integrator1/1 -> Damping/1, Speed/1, Ke/1
  (Inductance)1/1 -> Discrete-Time Integrator1/1
  Add1/1 -> (Inductance)1/1
  Kt/1 -> Add1/1
  Ke/1 -> Add/3
  Resistance/1 -> Add/1
  Discrete-Time Integrator/1 -> Resistance/1, Kt/1
  Add/1 -> (Inductance)/1
  Voltage/1 -> Add/2
  input/1 -> Voltage/1

== system c00019M_harness/M004/Physical/W5/DC_Engine ==
  input : Inport
  (Inductance) : Gain  Gain=1/L
  (Inductance)1 : Gain  Gain=1/J
  Add : Sum  Inputs=-+-
  Add1 : Sum  Inputs=+-
  Damping : Gain  Gain=b
  Discrete-Time Integrator : DiscreteIntegrator  SampleTime=-1  ICPrevOutput=DiscIntNeverNeededParam  ICPrevScaledInput=DiscIntNeverNeededParam
  Discrete-Time Integrator1 : DiscreteIntegrator  SampleTime=-1  ICPrevOutput=DiscIntNeverNeededParam  ICPrevScaledInput=DiscIntNeverNeededParam
  Ke : Gain  Gain=K
  Kt : Gain  Gain=K
  Resistance : Gain  Gain=R
  Voltage : Gain  Gain=10
  Speed : Outport
  wires:
  input/1 -> Voltage/1
  Voltage/1 -> Add/2
  Add/1 -> (Inductance)/1
  (Inductance)/1 -> Discrete-Time Integrator/1
  Discrete-Time Integrator/1 -> Kt/1, Resistance/1
  Resistance/1 -> Add/1
  Ke/1 -> Add/3
  Kt/1 -> Add1/1
  Add1/1 -> (Inductance)1/1
  (Inductance)1/1 -> Discrete-Time Integrator1/1
  Discrete-Time Integrator1/1 -> Ke/1, Speed/1, Damping/1
  Damping/1 -> Add1/2

== system c00019M_harness/M004/Physical/W7/DC_Engine ==
  input : Inport
  (Inductance) : Gain  Gain=1/L
  (Inductance)1 : Gain  Gain=1/J
  Add : Sum  Inputs=-+-
  Add1 : Sum  Inputs=+-
  Damping : Gain  Gain=b
  Discrete-Time Integrator : DiscreteIntegrator  SampleTime=-1  ICPrevOutput=DiscIntNeverNeededParam  ICPrevScaledInput=DiscIntNeverNeededParam
  Discrete-Time Integrator1 : DiscreteIntegrator  SampleTime=-1  ICPrevOutput=DiscIntNeverNeededParam  ICPrevScaledInput=DiscIntNeverNeededParam
  Ke : Gain  Gain=K
  Kt : Gain  Gain=K
  Resistance : Gain  Gain=R
  Voltage : Gain  Gain=10
  Speed : Outport
  wires:
  input/1 -> Voltage/1
  Voltage/1 -> Add/2
  Add/1 -> (Inductance)/1
  (Inductance)/1 -> Discrete-Time Integrator/1
  Discrete-Time Integrator/1 -> Kt/1, Resistance/1
  Resistance/1 -> Add/1
  Ke/1 -> Add/3
  Kt/1 -> Add1/1
  Add1/1 -> (Inductance)1/1
  (Inductance)1/1 -> Discrete-Time Integrator1/1
  Discrete-Time Integrator1/1 -> Ke/1, Speed/1, Damping/1
  Damping/1 -> Add1/2

== system c00019M_harness/M014/Physical/W/DC_Engine ==
  input : Inport
  (Inductance) : Gain  Gain=1/L
  (Inductance)1 : Gain  Gain=1/J
  Add : Sum  Inputs=-+-
  Add1 : Sum  Inputs=+-
  Damping : Gain  Gain=b
  Discrete-Time Integrator : DiscreteIntegrator  SampleTime=-1  ICPrevOutput=DiscIntNeverNeededParam  ICPrevScaledInput=DiscIntNeverNeededParam
  Discrete-Time Integrator1 : DiscreteIntegrator  SampleTime=-1  ICPrevOutput=DiscIntNeverNeededParam  ICPrevScaledInput=DiscIntNeverNeededParam
  Ke : Gain  Gain=K
  Kt : Gain  Gain=K
  Resistance : Gain  Gain=R
  Voltage : Gain  Gain=10
  Speed : Outport
  wires:
  (Inductance)/1 -> Discrete-Time Integrator/1
  Damping/1 -> Add1/2
  Discrete-Time Integrator1/1 -> Damping/1, Speed/1, Ke/1
  (Inductance)1/1 -> Discrete-Time Integrator1/1
  Add1/1 -> (Inductance)1/1
  Kt/1 -> Add1/1
  Ke/1 -> Add/3
  Resistance/1 -> Add/1
  Discrete-Time Integrator/1 -> Resistance/1, Kt/1
  Add/1 -> (Inductance)/1
  Voltage/1 -> Add/2
  input/1 -> Voltage/1

== system c00019M_harness/M014/Physical/W5/DC_Engine ==
  input : Inport
  (Inductance) : Gain  Gain=1/L
  (Inductance)1 : Gain  Gain=1/J
  Add : Sum  Inputs=-+-
  Add1 : Sum  Inputs=+-
  Damping : Gain  Gain=b
  Discrete-Time Integrator : DiscreteIntegrator  SampleTime=-1  ICPrevOutput=DiscIntNeverNeededParam  ICPrevScaledInput=DiscIntNeverNeededParam
  Discrete-Time Integrator1 : DiscreteIntegrator  SampleTime=-1  ICPrevOutput=DiscIntNeverNeededParam  ICPrevScaledInput=DiscIntNeverNeededParam
  Ke : Gain  Gain=K
  Kt : Gain  Gain=K
  Resistance : Gain  Gain=R
  Voltage : Gain  Gain=10
  Speed : Outport
  wires:
  input/1 -> Voltage/1
  Voltage/1 -> Add/2
  Add/1 -> (Inductance)/1
  (Inductance)/1 -> Discrete-Time Integrator/1
  Discrete-Time Integrator/1 -> Kt/1, Resistance/1
  Resistance/1 -> Add/1
  Ke/1 -> Add/3
  Kt/1 -> Add1/1
  Add1/1 -> (Inductance)1/1
  (Inductance)1/1 -> Discrete-Time Integrator1/1
  Discrete-Time Integrator1/1 -> Ke/1, Speed/1, Damping/1
  Damping/1 -> Add1/2

== system c00019M_harness/M014/Physical/W7/DC_Engine ==
  input : Inport
  (Inductance) : Gain  Gain=1/L
  (Inductance)1 : Gain  Gain=1/J
  Add : Sum  Inputs=-+-
  Add1 : Sum  Inputs=+-
  Damping : Gain  Gain=b
  Discrete-Time Integrator : DiscreteIntegrator  SampleTime=-1  ICPrevOutput=DiscIntNeverNeededParam  ICPrevScaledInput=DiscIntNeverNeededParam
  Discrete-Time Integrator1 : DiscreteIntegrator  SampleTime=-1  ICPrevOutput=DiscIntNeverNeededParam  ICPrevScaledInput=DiscIntNeverNeededParam
  Ke : Gain  Gain=K
  Kt : Gain  Gain=K
  Resistance : Gain  Gain=R
  Voltage : Gain  Gain=10
  Speed : Outport
  wires:
  input/1 -> Voltage/1
  Voltage/1 -> Add/2
  Add/1 -> (Inductance)/1
  (Inductance)/1 -> Discrete-Time Integrator/1
  Discrete-Time Integrator/1 -> Kt/1, Resistance/1
  Resistance/1 -> Add/1
  Ke/1 -> Add/3
  Kt/1 -> Add1/1
  Add1/1 -> (Inductance)1/1
  (Inductance)1/1 -> Discrete-Time Integrator1/1
  Discrete-Time Integrator1/1 -> Ke/1, Speed/1, Damping/1
  Damping/1 -> Add1/2

== system c00019M_harness/M018/Physical/W/DC_Engine ==
  input : Inport
  (Inductance) : Gain  Gain=1/L
  (Inductance)1 : Gain  Gain=1/J
  Add : Sum  Inputs=-+-
  Add1 : Sum  Inputs=+-
  Damping : Gain  Gain=b
  Discrete-Time Integrator : DiscreteIntegrator  SampleTime=-1  ICPrevOutput=DiscIntNeverNeededParam  ICPrevScaledInput=DiscIntNeverNeededParam
  Discrete-Time Integrator1 : DiscreteIntegrator  SampleTime=-1  ICPrevOutput=DiscIntNeverNeededParam  ICPrevScaledInput=DiscIntNeverNeededParam
  Ke : Gain  Gain=K
  Kt : Gain  Gain=K
  Resistance : Gain  Gain=R
  Voltage : Gain  Gain=10
  Speed : Outport
  wires:
  (Inductance)/1 -> Discrete-Time Integrator/1
  Damping/1 -> Add1/2
  Discrete-Time Integrator1/1 -> Damping/1, Speed/1, Ke/1
  (Inductance)1/1 -> Discrete-Time Integrator1/1
  Add1/1 -> (Inductance)1/1
  Kt/1 -> Add1/1
  Ke/1 -> Add/3
  Resistance/1 -> Add/1
  Discrete-Time Integrator/1 -> Resistance/1, Kt/1
  Add/1 -> (Inductance)/1
  Voltage/1 -> Add/2
  input/1 -> Voltage/1

== system c00019M_harness/M018/Physical/W5/DC_Engine ==
  input : Inport
  (Inductance) : Gain  Gain=1/L
  (Inductance)1 : Gain  Gain=1/J
  Add : Sum  Inputs=-+-
  Add1 : Sum  Inputs=+-
  Damping : Gain  Gain=b
  Discrete-Time Integrator : DiscreteIntegrator  SampleTime=-1  ICPrevOutput=DiscIntNeverNeededParam  ICPrevScaledInput=DiscIntNeverNeededParam
  Discrete-Time Integrator1 : DiscreteIntegrator  SampleTime=-1  ICPrevOutput=DiscIntNeverNeededParam  ICPrevScaledInput=DiscIntNeverNeededParam
  Ke : Gain  Gain=K
  Kt : Gain  Gain=K
  Resistance : Gain  Gain=R
  Voltage : Gain  Gain=10
  Speed : Outport
  wires:
  input/1 -> Voltage/1
  Voltage/1 -> Add/2
  Add/1 -> (Inductance)/1
  (Inductance)/1 -> Discrete-Time Integrator/1
  Discrete-Time Integrator/1 -> Kt/1, Resistance/1
  Resistance/1 -> Add/1
  Ke/1 -> Add/3
  Kt/1 -> Add1/1
  Add1/1 -> (Inductance)1/1
  (Inductance)1/1 -> Discrete-Time Integrator1/1
  Discrete-Time Integrator1/1 -> Ke/1, Speed/1, Damping/1
  Damping/1 -> Add1/2

== system c00019M_harness/M018/Physical/W7/DC_Engine ==
  input : Inport
  (Inductance) : Gain  Gain=1/L
  (Inductance)1 : Gain  Gain=1/J
  Add : Sum  Inputs=-+-
  Add1 : Sum  Inputs=+-
  Damping : Gain  Gain=b
  Discrete-Time Integrator : DiscreteIntegrator  SampleTime=-1  ICPrevOutput=DiscIntNeverNeededParam  ICPrevScaledInput=DiscIntNeverNeededParam
  Discrete-Time Integrator1 : DiscreteIntegrator  SampleTime=-1  ICPrevOutput=DiscIntNeverNeededParam  ICPrevScaledInput=DiscIntNeverNeededParam
  Ke : Gain  Gain=K
  Kt : Gain  Gain=K
  Resistance : Gain  Gain=R
  Voltage : Gain  Gain=10
  Speed : Outport
  wires:
  input/1 -> Voltage/1
  Voltage/1 -> Add/2
  Add/1 -> (Inductance)/1
  (Inductance)/1 -> Discrete-Time Integrator/1
  Discrete-Time Integrator/1 -> Kt/1, Resistance/1
  Resistance/1 -> Add/1
  Ke/1 -> Add/3
  Kt/1 -> Add1/1
  Add1/1 -> (Inductance)1/1
  (Inductance)1/1 -> Discrete-Time Integrator1/1
  Discrete-Time Integrator1/1 -> Ke/1, Speed/1, Damping/1
  Damping/1 -> Add1/2

== system c00019M_harness/M028/Physical/W/DC_Engine ==
  input : Inport
  (Inductance) : Gain  Gain=1/L
  (Inductance)1 : Gain  Gain=1/J
  Add : Sum  Inputs=-+-
  Add1 : Sum  Inputs=+-
  Damping : Gain  Gain=b
  Discrete-Time Integrator : DiscreteIntegrator  SampleTime=-1  ICPrevOutput=DiscIntNeverNeededParam  ICPrevScaledInput=DiscIntNeverNeededParam
  Discrete-Time Integrator1 : DiscreteIntegrator  SampleTime=-1  ICPrevOutput=DiscIntNeverNeededParam  ICPrevScaledInput=DiscIntNeverNeededParam
  Ke : Gain  Gain=K
  Kt : Gain  Gain=K
  Resistance : Gain  Gain=R
  Voltage : Gain  Gain=10
  Speed : Outport
  wires:
  (Inductance)/1 -> Discrete-Time Integrator/1
  Damping/1 -> Add1/2
  Discrete-Time Integrator1/1 -> Damping/1, Speed/1, Ke/1
  (Inductance)1/1 -> Discrete-Time Integrator1/1
  Add1/1 -> (Inductance)1/1
  Kt/1 -> Add1/1
  Ke/1 -> Add/3
  Resistance/1 -> Add/1
  Discrete-Time Integrator/1 -> Resistance/1, Kt/1
  Add/1 -> (Inductance)/1
  Voltage/1 -> Add/2
  input/1 -> Voltage/1

== system c00019M_harness/M028/Physical/W5/DC_Engine ==
  input : Inport
  (Inductance) : Gain  Gain=1/L
  (Inductance)1 : Gain  Gain=1/J
  Add : Sum  Inputs=-+-
  Add1 : Sum  Inputs=+-
  Damping : Gain  Gain=b
  Discrete-Time Integrator : DiscreteIntegrator  SampleTime=-1  ICPrevOutput=DiscIntNeverNeededParam  ICPrevScaledInput=DiscIntNeverNeededParam
  Discrete-Time Integrator1 : DiscreteIntegrator  SampleTime=-1  ICPrevOutput=DiscIntNeverNeededParam  ICPrevScaledInput=DiscIntNeverNeededParam
  Ke : Gain  Gain=K
  Kt : Gain  Gain=K
  Resistance : Gain  Gain=R
  Voltage : Gain  Gain=10
  Speed : Outport
  wires:
  input/1 -> Voltage/1
  Voltage/1 -> Add/2
  Add/1 -> (Inductance)/1
  (Inductance)/1 -> Discrete-Time Integrator/1
  Discrete-Time Integrator/1 -> Kt/1, Resistance/1
  Resistance/1 -> Add/1
  Ke/1 -> Add/3
  Kt/1 -> Add1/1
  Add1/1 -> (Inductance)1/1
  (Inductance)1/1 -> Discrete-Time Integrator1/1
  Discrete-Time Integrator1/1 -> Ke/1, Speed/1, Damping/1
  Damping/1 -> Add1/2

== system c00019M_harness/M028/Physical/W7/DC_Engine ==
  input : Inport
  (Inductance) : Gain  Gain=1/L
  (Inductance)1 : Gain  Gain=1/J
  Add : Sum  Inputs=-+-
  Add1 : Sum  Inputs=+-
  Damping : Gain  Gain=b
  Discrete-Time Integrator : DiscreteIntegrator  SampleTime=-1  ICPrevOutput=DiscIntNeverNeededParam  ICPrevScaledInput=DiscIntNeverNeededParam
  Discrete-Time Integrator1 : DiscreteIntegrator  SampleTime=-1  ICPrevOutput=DiscIntNeverNeededParam  ICPrevScaledInput=DiscIntNeverNeededParam
  Ke : Gain  Gain=K
  Kt : Gain  Gain=K
  Resistance : Gain  Gain=R
  Voltage : Gain  Gain=10
  Speed : Outport
  wires:
  input/1 -> Voltage/1
  Voltage/1 -> Add/2
  Add/1 -> (Inductance)/1
  (Inductance)/1 -> Discrete-Time Integrator/1
  Discrete-Time Integrator/1 -> Kt/1, Resistance/1
  Resistance/1 -> Add/1
  Ke/1 -> Add/3
  Kt/1 -> Add1/1
  Add1/1 -> (Inductance)1/1
  (Inductance)1/1 -> Discrete-Time Integrator1/1
  Discrete-Time Integrator1/1 -> Ke/1, Speed/1, Damping/1
  Damping/1 -> Add1/2

== system c00019M_harness/M033/Physical/W/DC_Engine ==
  input : Inport
  (Inductance) : Gain  Gain=1/L
  (Inductance)1 : Gain  Gain=1/J
  Add : Sum  Inputs=-+-
  Add1 : Sum  Inputs=+-
  Damping : Gain  Gain=b
  Discrete-Time Integrator : DiscreteIntegrator  SampleTime=-1  ICPrevOutput=DiscIntNeverNeededParam  ICPrevScaledInput=DiscIntNeverNeededParam
  Discrete-Time Integrator1 : DiscreteIntegrator  SampleTime=-1  ICPrevOutput=DiscIntNeverNeededParam  ICPrevScaledInput=DiscIntNeverNeededParam
  Ke : Gain  Gain=K
  Kt : Gain  Gain=K
  Resistance : Gain  Gain=R
  Voltage : Gain  Gain=10
  Speed : Outport
  wires:
  (Inductance)/1 -> Discrete-Time Integrator/1
  Damping/1 -> Add1/2
  Discrete-Time Integrator1/1 -> Damping/1, Speed/1, Ke/1
  (Inductance)1/1 -> Discrete-Time Integrator1/1
  Add1/1 -> (Inductance)1/1
  Kt/1 -> Add1/1
  Ke/1 -> Add/3
  Resistance/1 -> Add/1
  Discrete-Time Integrator/1 -> Resistance/1, Kt/1
  Add/1 -> (Inductance)/1
  Voltage/1 -> Add/2
  input/1 -> Voltage/1

== system c00019M_harness/M033/Physical/W5/DC_Engine ==
  input : Inport
  (Inductance) : Gain  Gain=1/L
  (Inductance)1 : Gain  Gain=1/J
  Add : Sum  Inputs=-+-
  Add1 : Sum  Inputs=+-
  Damping : Gain  Gain=b
  Discrete-Time Integrator : DiscreteIntegrator  SampleTime=-1  ICPrevOutput=DiscIntNeverNeededParam  ICPrevScaledInput=DiscIntNeverNeededParam
  Discrete-Time Integrator1 : DiscreteIntegrator  SampleTime=-1  ICPrevOutput=DiscIntNeverNeededParam  ICPrevScaledInput=DiscIntNeverNeededParam
  Ke : Gain  Gain=K
  Kt : Gain  Gain=K
  Resistance : Gain  Gain=R
  Voltage : Gain  Gain=10
  Speed : Outport
  wires:
  input/1 -> Voltage/1
  Voltage/1 -> Add/2
  Add/1 -> (Inductance)/1
  (Inductance)/1 -> Discrete-Time Integrator/1
  Discrete-Time Integrator/1 -> Kt/1, Resistance/1
  Resistance/1 -> Add/1
  Ke/1 -> Add/3
  Kt/1 -> Add1/1
  Add1/1 -> (Inductance)1/1
  (Inductance)1/1 -> Discrete-Time Integrator1/1
  Discrete-Time Integrator1/1 -> Ke/1, Speed/1, Damping/1
  Damping/1 -> Add1/2

== system c00019M_harness/M033/Physical/W7/DC_Engine ==
  input : Inport
  (Inductance) : Gain  Gain=1/L
  (Inductance)1 : Gain  Gain=1/J
  Add : Sum  Inputs=-+-
  Add1 : Sum  Inputs=+-
  Damping : Gain  Gain=b
  Discrete-Time Integrator : DiscreteIntegrator  SampleTime=-1  ICPrevOutput=DiscIntNeverNeededParam  ICPrevScaledInput=DiscIntNeverNeededParam
  Discrete-Time Integrator1 : DiscreteIntegrator  SampleTime=-1  ICPrevOutput=DiscIntNeverNeededParam  ICPrevScaledInput=DiscIntNeverNeededParam
  Ke : Gain  Gain=K
  Kt : Gain  Gain=K
  Resistance : Gain  Gain=R
  Voltage : Gain  Gain=10
  Speed : Outport
  wires:
  input/1 -> Voltage/1
  Voltage/1 -> Add/2
  Add/1 -> (Inductance)/1
  (Inductance)/1 -> Discrete-Time Integrator/1
  Discrete-Time Integrator/1 -> Kt/1, Resistance/1
  Resistance/1 -> Add/1
  Ke/1 -> Add/3
  Kt/1 -> Add1/1
  Add1/1 -> (Inductance)1/1
  (Inductance)1/1 -> Discrete-Time Integrator1/1
  Discrete-Time Integrator1/1 -> Ke/1, Speed/1, Damping/1
  Damping/1 -> Add1/2

== system c00019M_harness/M043/Physical/W/DC_Engine ==
  input : Inport
  (Inductance) : Gain  Gain=1/L
  (Inductance)1 : Gain  Gain=1/J
  Add : Sum  Inputs=-+-
  Add1 : Sum  Inputs=+-
  Damping : Gain  Gain=b
  Discrete-Time Integrator : DiscreteIntegrator  SampleTime=-1  ICPrevOutput=DiscIntNeverNeededParam  ICPrevScaledInput=DiscIntNeverNeededParam
  Discrete-Time Integrator1 : DiscreteIntegrator  SampleTime=-1  ICPrevOutput=DiscIntNeverNeededParam  ICPrevScaledInput=DiscIntNeverNeededParam
  Ke : Gain  Gain=K
  Kt : Gain  Gain=K
  Resistance : Gain  Gain=R
  Voltage : Gain  Gain=10
  Speed : Outport
  wires:
  (Inductance)/1 -> Discrete-Time Integrator/1
  Damping/1 -> Add1/2
  Discrete-Time Integrator1/1 -> Damping/1, Speed/1, Ke/1
  (Inductance)1/1 -> Discrete-Time Integrator1/1
  Add1/1 -> (Inductance)1/1
  Kt/1 -> Add1/1
  Ke/1 -> Add/3
  Resistance/1 -> Add/1
  Discrete-Time Integrator/1 -> Resistance/1, Kt/1
  Add/1 -> (Inductance)/1
  Voltage/1 -> Add/2
  input/1 -> Voltage/1
